simulink model "sm_ik_trajectory"  (R2023a)
settings: Solver=VariableStepAuto  StartTime=0.0  StopTime=10  RelTol=1e-3
values from neighbouring files (symbols this model uses):
  n = dims(1)    [RunMyCobot.m]
libraries: simulink x3, robotcorelib x1, robotmaniplib x1
settings Model: Creator=The MathWorks, Inc.  LastModifiedBy=yoganandam
settings SolverCC: AlgebraicLoopSolver=TrustRegion
settings DataIOCC: ReturnWorkspaceOutputs=off
settings DebuggingCC: UnconnectedInputMsg=warning  UnconnectedOutputMsg=warning  UnconnectedLineMsg=warning  ArithmeticOperatorsInVariantConditions=warning
settings ModelReferenceCC: EnableRefExpFcnMdlSchedulingChecks=on
settings SFSimCC: SimUseLocalCustomCode=off  CustomCodeUndefinedFunction=UseInterfaceOnly
settings RTWCC: RTWUseLocalCustomCode=off

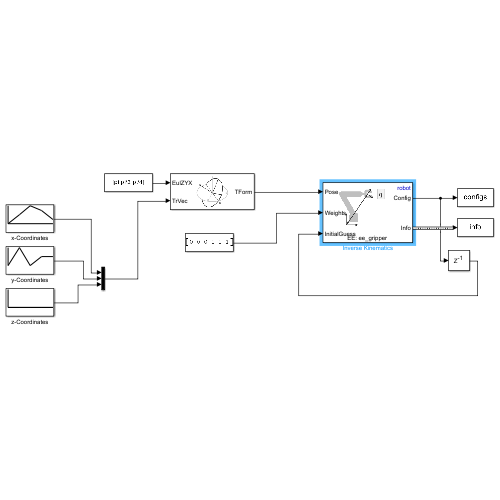
[thumbnail: Simulink's stored preview of the top-level diagram]
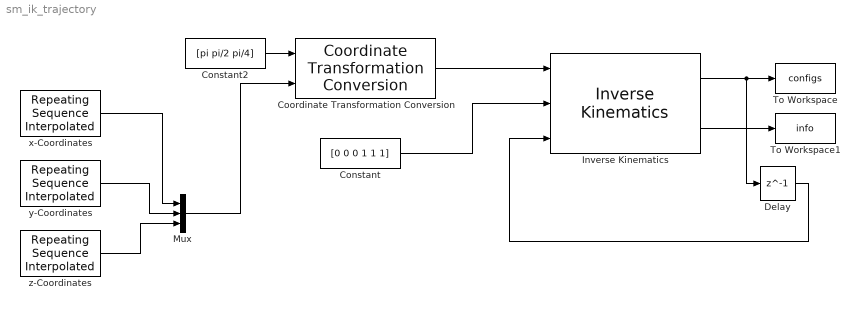
== system sm_ik_trajectory ==
  Constant : Constant  Value=[0 0 0 1 1 1]  VectorParams1D=off
  Constant2 : Constant  Value=[pi pi/2 pi/4]
  Coordinate Transformation Conversion : robotcorelib/Coordinate Transformation Conversion  InputRepresentation=Euler Angles  InputEulerSequence=ZYX  ShowTrVecInputPort=on  OutputRepresentation=Homogeneous Transformation  OutputEulerSequence=ZYX  ShowTrVecOutputPort=on  SimulateUsing=Interpreted execution
  Delay : Delay  DelayLength=1  InitialCondition=zeros(6,1)
  Inverse Kinematics : robotmaniplib/Inverse Kinematics  RigidBodyTree=robot  EndEffector=ee_gripper  ShowInfo=on  SolverName=BFGS Gradient Projection  EnforceJointLimits=on  MaxIterations=1500  MaxTime=10  GradientTolerance=1e-5  SolutionTolerance=1e-4  StepTolerance=1e-10  ErrorChangeTolerance=1e-12  UseErrorDamping=on  DampingBias=0.0025  SimulateUsing=Interpreted execution
  Mux : Mux  Inputs=3
  To Workspace : ToWorkspace  VariableName=configs  SaveFormat=Timeseries  SampleTime=-1
  To Workspace1 : ToWorkspace  VariableName=info  SaveFormat=Timeseries  SampleTime=-1
  "x-Coordinates " : simulink/Sources/Repeating Sequence Interpolated  OutValues=x  TimeValues=linspace(0,10,n)  LookUpMeth=Interpolation-Use End Values  tsamp=time_step  OutMin=[]  OutMax=[]  OutDataTypeStr=double  OutputDataTypeScalingMode=double  OutDataType=fixdt(0,8)  OutScaling=2^-10
  y-Coordinates : simulink/Sources/Repeating Sequence Interpolated  OutValues=y  TimeValues=linspace(0,10,n)  LookUpMeth=Interpolation-Use End Values  tsamp=time_step  OutMin=[]  OutMax=[]  OutDataTypeStr=double  OutputDataTypeScalingMode=double  OutDataType=fixdt(0,8)  OutScaling=2^-10
  z-Coordinates : simulink/Sources/Repeating Sequence Interpolated  OutValues=z  TimeValues=linspace(0,10,n)  LookUpMeth=Interpolation-Use End Values  tsamp=time_step  OutMin=[]  OutMax=[]  OutDataTypeStr=double  OutputDataTypeScalingMode=double  OutDataType=fixdt(0,8)  OutScaling=2^-10
  wires:
  "x-Coordinates "/1 -> Mux/1
  Coordinate Transformation Conversion/1 -> Inverse Kinematics/1
  Mux/1 -> Coordinate Transformation Conversion/2
  y-Coordinates/1 -> Mux/2
  z-Coordinates/1 -> Mux/3
  Constant/1 -> Inverse Kinematics/2
  Inverse Kinematics/1 -> Delay/1, To Workspace/1
  Inverse Kinematics/2 -> To Workspace1/1
  Delay/1 -> Inverse Kinematics/3
  Constant2/1 -> Coordinate Transformation Conversion/1
